simulink model "FuzzyRaspberry"  (R2017b)
settings: Solver=VariableStepAuto  StartTime=0.0  StopTime=800  RelTol=1e-3
libraries: fuzblock x1
settings Model: Creator=Eneko  LastModifiedBy=Eneko

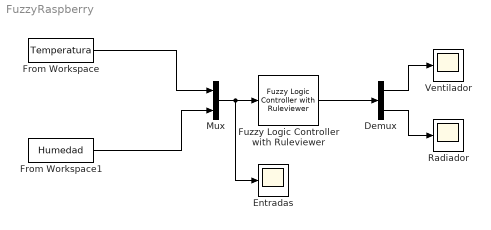
== system FuzzyRaspberry ==
  Demux : Demux  Outputs=2
  Entradas : Scope
  From Workspace : FromWorkspace  VariableName=Temperatura  SampleTime=0
  From Workspace1 : FromWorkspace  VariableName=Humedad  SampleTime=0
  Fuzzy Logic Controller with Ruleviewer : fuzblock/Fuzzy Logic  Controller  with Ruleviewer  fismatrix=FuzzyRaspberry  Ts=10
  Mux : Mux  Inputs=2
  Radiador : Scope
  Ventilador : Scope
  wires:
  Mux/1 -> Entradas/1, Fuzzy Logic Controller with Ruleviewer/1
  From Workspace/1 -> Mux/1
  From Workspace1/1 -> Mux/2
  Fuzzy Logic Controller with Ruleviewer/1 -> Demux/1
  Demux/1 -> Ventilador/1
  Demux/2 -> Radiador/1
